simulink model "HoverQuadmodel_with_LQR_controller"  (R2021a)
settings: Solver=VariableStepAuto  StartTime=0.0  StopTime=10.0  RelTol=1e-3
values from neighbouring files (symbols this model uses):
  A = [0 0 0 1 0 0;0 0 0 0 1 0;0 0 0 0 0 1;0 0 0 0 0 0;0 0 0 0 0 0;0 0 0 0 0 0]    [Statematrix.m]    (also in parameter.m)
  B = [0 0 0 0;0 0 0 0;0 0 0 0;-kt/jy -kt/jy kt/jy kt/jy;L*kf/jp -L*kf/jp 0 0;0 0 L*kf/jr -L*kf/jr]    [Statematrix.m]    (also in parameter.m)
  C = [1 0 0 0 0 0;0 1 0 0 0 0;0 0 1 0 0 0]    [Statematrix.m]    (also in parameter.m)
  D = [0 0 0 0;0 0 0 0;0 0 0 0]    [Statematrix.m]    (also in parameter.m)
  K_LQR = [-111.8 132.3 0 -41.41 36.23 0;-111.8 -132.3 0 -41.41 -36.23 0;111.8 0 132.3 41.41 0 36.23;111.8 0 -132.3 41.41 0 -36.23]    [parameter.m]
  V_bias = 2    [parameter.m]
  VMAX_AMP = 24    [parameter.m]
undefined symbols (not defined in the file or in its folder): sigbuilder_block
libraries: simulink_extras x4
settings Model: Creator=44743  LastModifiedBy=44743

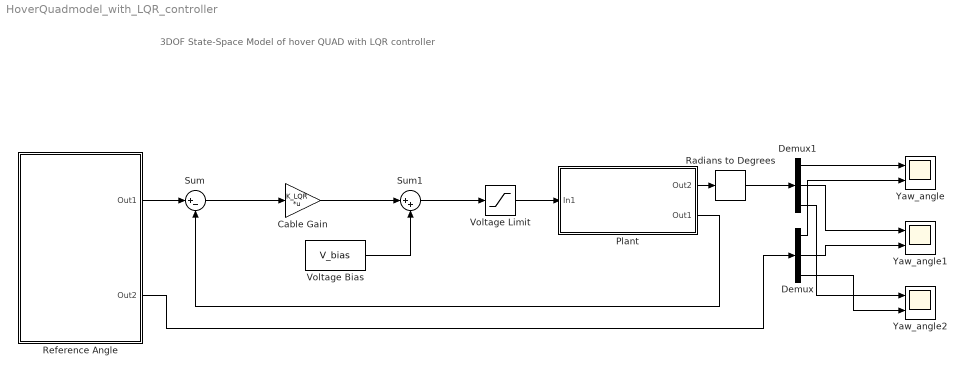
== system HoverQuadmodel_with_LQR_controller ==
  note: 3DOF State-Space Model of hover QUAD with LQR controller
  Cable Gain : Gain  Gain=K_LQR  Multiplication=Matrix(K*u)  SaturateOnIntegerOverflow=on  OutDataTypeStr=Inherit: Same as input  ParamDataTypeStr=Inherit: Same as input
  Demux : Demux  Outputs=3
  Demux1 : Demux  Outputs=3
  Plant : Subsystem
  Radians to Degrees : simulink_extras/Transformations/Radians to Degrees
  Reference Angle : Subsystem
  Sum : Sum  Inputs=|+-
  Sum1 : Sum  Inputs=|++
  Voltage Bias : Constant  Value=V_bias
  Voltage Limit : Saturate  UpperLimit=VMAX_AMP  LowerLimit=0
  Yaw_angle : Scope  NumInputPorts=2
  Yaw_angle1 : Scope  NumInputPorts=2
  Yaw_angle2 : Scope  NumInputPorts=2
  wires:
  Cable Gain/1 -> Sum1/1
  Voltage Bias/1 -> Sum1/2
  Sum/1 -> Cable Gain/1
  Sum1/1 -> Voltage Limit/1
  Voltage Limit/1 -> Plant/1(In1)
  Plant/2(Out1) -> Sum/2
  Plant/1(Out2) -> Radians to Degrees/1
  Radians to Degrees/1 -> Demux1/1
  Reference Angle/1(Out1) -> Sum/1
  Reference Angle/2(Out2) -> Demux/1
  Demux1/1 -> Yaw_angle/1
  Demux/1 -> Yaw_angle/2
  Demux1/2 -> Yaw_angle1/1
  Demux/2 -> Yaw_angle1/2
  Demux1/3 -> Yaw_angle2/1
  Demux/3 -> Yaw_angle2/2

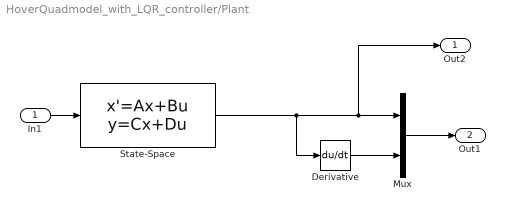
== system HoverQuadmodel_with_LQR_controller/Plant ==
  In1 : Inport
  Derivative : Derivative
  Mux : Mux  Inputs=2
  State-Space : StateSpace  A=A  B=B  C=C  D=D  InitialCondition=0
  Out2 : Outport
  Out1 : Outport  Port=2
  wires:
  In1/1 -> State-Space/1
  State-Space/1 -> Derivative/1, Out2/1, Mux/1
  Derivative/1 -> Mux/2
  Mux/1 -> Out1/1

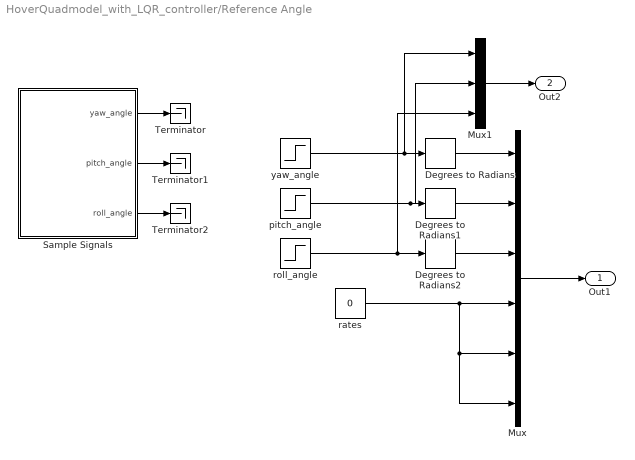
== system HoverQuadmodel_with_LQR_controller/Reference Angle ==
  Degrees to Radians : simulink_extras/Transformations/Degrees to Radians
  Degrees to Radians1 : simulink_extras/Transformations/Degrees to Radians
  Degrees to Radians2 : simulink_extras/Transformations/Degrees to Radians
  Mux : Mux  Inputs=6
  Mux1 : Mux  Inputs=3
  Sample Signals : Subsystem  Tag=STV Subsys  LoadFcn=sigbuilder_block('load');  StartFcn=sigbuilder_block('start');  StopFcn=sigbuilder_block('stop');  ClipboardFcn=sigbuilder_block('clipboard');  mask(Sigbuilder block){tuvar=[0:10]}
      mask help: Simulink:masks:SigbuilderBlock_MD
      mask init:
      | if ~strcmp(get_param(bdroot(gcbh),'SimulationStatus'),'stopped') tuvar = sigbuilder_block('maskInit'); end
      settings: CopyFcn=sigbuilder_block('copy');  DeleteFcn=sigbuilder_block('delete');  ModelCloseFcn=sigbuilder_block('modelClose');  PreSaveFcn=sigbuilder_block('preSave');  PauseFcn=sigbuilder_block('pause');  ContinueFcn=sigbuilder_block('continue');  NameChangeFcn=sigbuilder_block('namechange');  OpenFcn=sigbuilder_block('open',[89.25 189 550.5 399.75 ]);  CloseFcn=sigbuilder_block('close');
      mask Display: plot(0, 0, 100, 100,[2, 2, 32, 32, 2], [68, 8, 8, 68, 68],[32, 2], [38, 38], [32, 19, 2],[53, 60, 44], [32, 17, 17, 2],[16, 16, 31, 31]);txt = getActiveGroup(gcbh);text(2, 100, txt,'verticalAlignment', 'top');
  Terminator : Terminator
  Terminator1 : Terminator
  Terminator2 : Terminator
  pitch_angle : Step  Time=2  SampleTime=0.1
  rates : Constant  Value=0
  roll_angle : Step  Time=2  SampleTime=0.08
  yaw_angle : Step  Time=5  SampleTime=0.04
  Out1 : Outport
  Out2 : Outport  Port=2
  wires:
  Degrees to Radians2/1 -> Mux/3
  Mux/1 -> Out1/1
  Degrees to Radians1/1 -> Mux/2
  Degrees to Radians/1 -> Mux/1
  rates/1 -> Mux/6, Mux/5, Mux/4
  yaw_angle/1 -> Mux1/1, Degrees to Radians/1
  pitch_angle/1 -> Mux1/2, Degrees to Radians1/1
  roll_angle/1 -> Degrees to Radians2/1, Mux1/3
  Mux1/1 -> Out2/1
  Sample Signals/1(yaw_angle) -> Terminator/1
  Sample Signals/2(pitch_angle) -> Terminator1/1
  Sample Signals/3(roll_angle) -> Terminator2/1

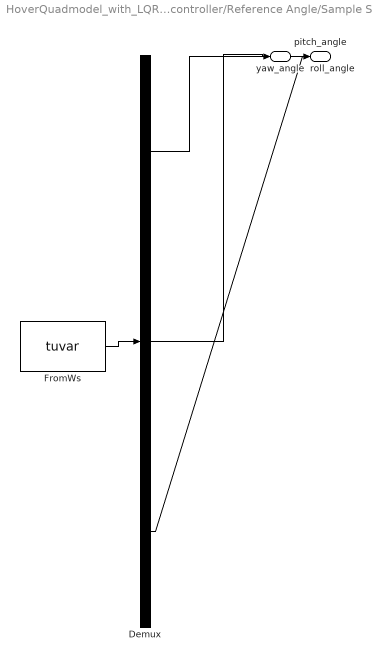
== system HoverQuadmodel_with_LQR_controller/Reference Angle/Sample Signals ==
  Demux : Demux  Tag=STV Demux  Outputs=3
      settings: DisplayOption=none
  FromWs : FromWorkspace  Tag=STV FromWs  VariableName=tuvar
      SigBuilderData=|
      | common.afterFinalStr = 'Extrapolate'
      | common.sampleTime = 0
      | dataSet.timeRange = [0 10]
      | dataSet.name = 'Group 1'
      | sbobj.Groups.Name = 'Group 1'
      | sbobj.Groups.Signals(1).Name = 'yaw_angle'
      | sbobj.Groups.Signals(1).XData = [0 7 7 8.62 8.62 10]
      | sbobj.Groups.Signals(1).YData = [0 0 1 1 0 0]
      | sbobj.Groups.Signals(2).Name = 'pitch_angle'
      | sbobj.Groups.Signals(2).XData = [0 1 1 3 3 10]
      | sbobj.Groups.Signals(2).YData = [0 0 1 1 0 0]
      | sbobj.Groups.Signals(3).Name = 'roll_angle'
      | sbobj.Groups.Signals(3).XData = [0 4 4 6 6 10]
      | sbobj.Groups.Signals(3).YData = [0 0 1 1 0 0]
  yaw_angle : Outport  Tag=STV Outport
  pitch_angle : Outport  Tag=STV Outport  Port=2
  roll_angle : Outport  Tag=STV Outport  Port=3
  wires:
  Demux/1 -> yaw_angle/1
  FromWs/1 -> Demux/1
  Demux/2 -> pitch_angle/1
  Demux/3 -> roll_angle/1
